simulink model "SMCsimplificado"  (R2020b)
settings: Solver=VariableStepAuto  StartTime=0.0  StopTime=10.0  MaxStep=0.02  RelTol=2e-3
undefined symbols (not defined in the file): a, B, beta, cond_init, d, delta, g, Go, J, Ke, Kt, m
settings Model: Creator=andre  LastModifiedBy=andre

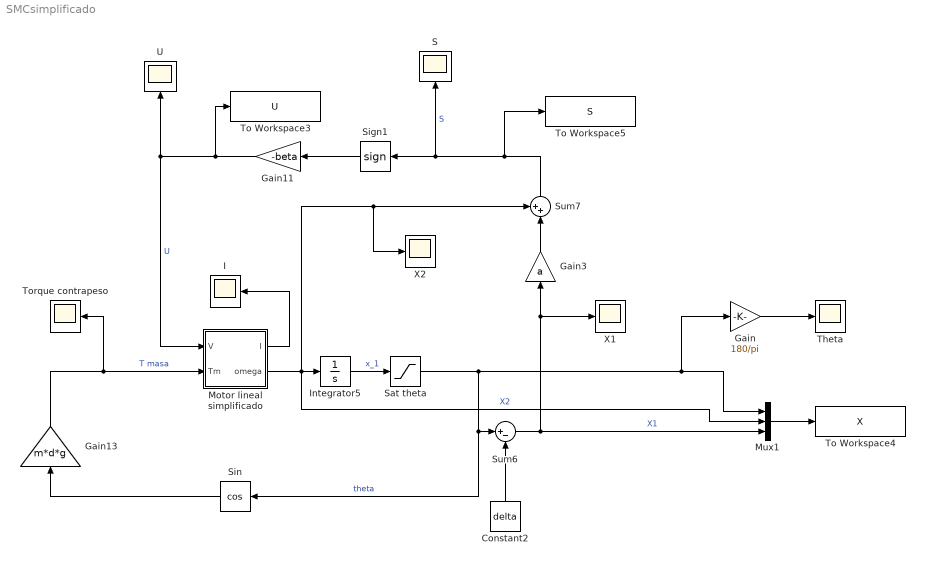
== system SMCsimplificado ==
  " Theta" : Scope
  Constant2 : Constant  Value=delta
  Gain : Gain  Gain=180/pi
  Gain11 : Gain  Gain=-beta
  Gain13 : Gain  Gain=m*d*g
  Gain3 : Gain  Gain=a
  I : Scope
  Integrator5 : Integrator  InitialCondition=cond_init
  Motor lineal simplificado : Subsystem
  Mux1 : Mux  Inputs=3
  S : Scope
  Sat theta : Saturate  UpperLimit=pi  LowerLimit=-pi
  Sign1 : Signum  ZeroCross=off
  Sin : Trigonometry  Operator=cos
  Sum6 : Sum  Inputs=|+-
  Sum7 : Sum  Inputs=++|
  To Workspace3 : ToWorkspace  VariableName=U  SaveFormat=Timeseries  SampleTime=-1
  To Workspace4 : ToWorkspace  VariableName=X  SaveFormat=Timeseries  SampleTime=-1
  To Workspace5 : ToWorkspace  VariableName=S  SaveFormat=Timeseries  SampleTime=-1
  Torque contrapeso : Scope
  U : Scope
  X1 : Scope
  X2 : Scope
  wires:
  Sat theta/1 -> Gain/1, Mux1/1, Sum6/1, Sin/1  "theta"
  Sum7/1 -> To Workspace5/1, S/1, Sign1/1  "S"
  Sum6/1 -> X1/1, Gain3/1, Mux1/3  "X1"
  Gain11/1 -> To Workspace3/1, Motor lineal simplificado/1(V), U/1  "U"
  Gain3/1 -> Sum7/2
  Mux1/1 -> To Workspace4/1
  Sin/1 -> Gain13/1
  Sign1/1 -> Gain11/1
  Integrator5/1 -> Sat theta/1  "x_1"
  Constant2/1 -> Sum6/2
  Gain13/1 -> Torque contrapeso/1, Motor lineal simplificado/2(Tm)  "T masa"
  Motor lineal simplificado/2(omega) -> Integrator5/1, Sum7/1, X2/1, Mux1/2  "X2"
  Motor lineal simplificado/1(I) -> I/1
  Gain/1 -> " Theta"/1

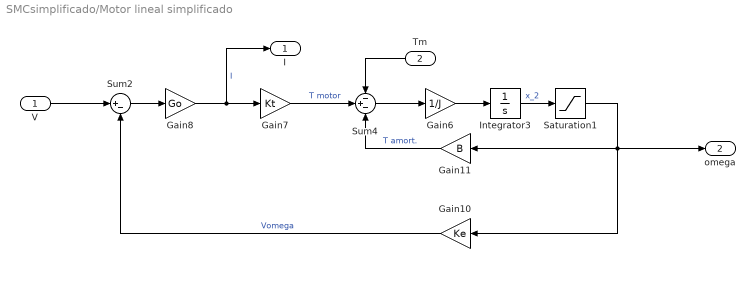
== system SMCsimplificado/Motor lineal simplificado ==
  V : Inport
  Tm : Inport  Port=2
  Gain10 : Gain  Gain=Ke
  Gain11 : Gain  Gain=B
  Gain6 : Gain  Gain=1/J
  Gain7 : Gain  Gain=Kt
  Gain8 : Gain  Gain=Go
  Integrator3 : Integrator
  Saturation1 : Saturate  UpperLimit=pi/2  LowerLimit=-pi/2
  Sum2 : Sum  Inputs=|+-
  Sum4 : Sum  Inputs=-+-
  I : Outport
  omega : Outport  Port=2
  wires:
  Gain10/1 -> Sum2/2  "Vomega"
  Sum4/1 -> Gain6/1
  Integrator3/1 -> Saturation1/1  "x_2"
  Gain11/1 -> Sum4/3  "T amort."
  Sum2/1 -> Gain8/1
  Gain7/1 -> Sum4/2  "T motor"
  Gain6/1 -> Integrator3/1
  Gain8/1 -> I/1, Gain7/1  "I"
  V/1 -> Sum2/1
  Tm/1 -> Sum4/1
  Saturation1/1 -> Gain11/1, Gain10/1, omega/1
